simulink model "lab6_5"  (R2018b)
settings: Solver=VariableStepAuto  StartTime=0.0  StopTime=10.0  RelTol=1e-3
libraries: hdlsllib x17
settings Model: Creator=mllax8  LastModifiedBy=mllax8

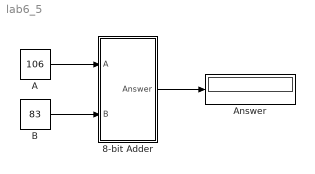
== system lab6_5 ==
  8-bit Adder : Subsystem
  A : Constant  Value=106  OutDataTypeStr=uint16
  Answer : Display
  B : Constant  Value=83  OutDataTypeStr=uint16
  wires:
  A/1 -> 8-bit Adder/1(A)
  B/1 -> 8-bit Adder/2(B)
  8-bit Adder/1(Answer) -> Answer/1

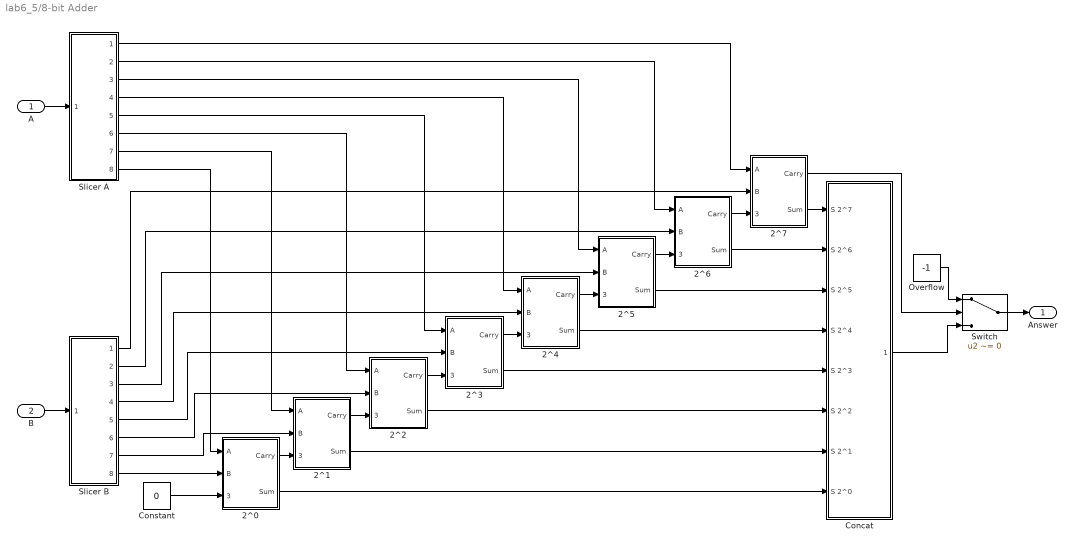
== system lab6_5/8-bit Adder ==
  A : Inport
  B : Inport  Port=2
  2^0 : Subsystem
  2^1 : Subsystem
  2^2 : Subsystem
  2^3 : Subsystem
  2^4 : Subsystem
  2^5 : Subsystem
  2^6 : Subsystem
  2^7 : Subsystem
  Concat : Subsystem
  Constant : Constant  Value=0
  Overflow : Constant  Value=-1  OutDataTypeStr=double
  Slicer A : Subsystem
  Slicer B : Subsystem
  Switch : Switch  Criteria=u2 ~= 0
  Answer : Outport
  wires:
  Slicer B/8("B 2^0 ") -> 2^0/2(B)
  2^7/2(Sum) -> Concat/1(S 2^7)
  Slicer B/5(B 2^3) -> 2^3/2(B)
  2^3/2(Sum) -> Concat/5(S 2^3)
  2^5/1(Carry) -> 2^6/3(Carry In)
  Slicer B/4(B 2^4) -> 2^4/2(B)
  Constant/1 -> 2^0/3(Carry In)
  2^4/2(Sum) -> Concat/4(S 2^4)
  Slicer B/6(B 2^2) -> 2^2/2(B)
  2^6/2(Sum) -> Concat/2(S 2^6)
  Slicer A/7(A 2^1) -> 2^1/1(A)
  2^4/1(Carry) -> 2^5/3(Carry In)
  2^5/2(Sum) -> Concat/3(S 2^5)
  2^3/1(Carry) -> 2^4/3(Carry In)
  Slicer B/1(B 2^7) -> 2^7/2(B)
  Slicer A/1(A 2^7) -> 2^7/1(A)
  2^1/1(Carry) -> 2^2/3(Carry In)
  2^0/1(Carry) -> 2^1/3(Carry In)
  Slicer B/3(B 2^5) -> 2^5/2(B)
  Slicer A/8("A 2^0 ") -> 2^0/1(A)
  2^0/2(Sum) -> Concat/8(S 2^0)
  Slicer A/5(A 2^3) -> 2^3/1(A)
  2^2/1(Carry) -> 2^3/3(Carry In)
  Slicer B/7(B 2^1) -> 2^1/2(B)
  Slicer A/4(A 2^4) -> 2^4/1(A)
  2^2/2(Sum) -> Concat/6(S 2^2)
  2^6/1(Carry) -> 2^7/3(Carry In)
  B/1 -> Slicer B/1(sign Int)
  Slicer A/2(A 2^6) -> 2^6/1(A)
  2^1/2(Sum) -> Concat/7(S 2^1)
  Slicer A/3(A 2^5) -> 2^5/1(A)
  Slicer B/2(B 2^6) -> 2^6/2(B)
  2^7/1(Carry) -> Switch/2
  Slicer A/6(A 2^2) -> 2^2/1(A)
  A/1 -> Slicer A/1(sign Int)
  Overflow/1 -> Switch/1
  Switch/1 -> Answer/1
  Concat/1(unsign Int) -> Switch/3

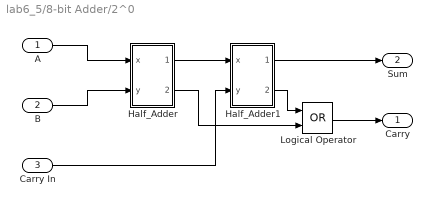
== system lab6_5/8-bit Adder/2^0 ==
  A : Inport
  B : Inport  Port=2
  Carry In : Inport  Port=3
  Half_Adder : Subsystem
  Half_Adder1 : Subsystem
  Logical Operator : Logic  Operator=OR  AllPortsSameDT=off  OutDataTypeStr=boolean
  Carry : Outport
  Sum : Outport  Port=2
  wires:
  Half_Adder1/1(Sum) -> Sum/1
  Carry In/1 -> Half_Adder1/2(y)
  Logical Operator/1 -> Carry/1
  Half_Adder1/2(Carry) -> Logical Operator/1
  A/1 -> Half_Adder/1(x)
  B/1 -> Half_Adder/2(y)
  Half_Adder/2(Carry) -> Logical Operator/2
  Half_Adder/1(Sum) -> Half_Adder1/1(x)

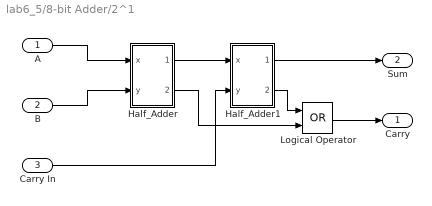
== system lab6_5/8-bit Adder/2^1 ==
  A : Inport
  B : Inport  Port=2
  Carry In : Inport  Port=3
  Half_Adder : Subsystem
  Half_Adder1 : Subsystem
  Logical Operator : Logic  Operator=OR  AllPortsSameDT=off  OutDataTypeStr=boolean
  Carry : Outport
  Sum : Outport  Port=2
  wires:
  Half_Adder1/1(Sum) -> Sum/1
  Carry In/1 -> Half_Adder1/2(y)
  Logical Operator/1 -> Carry/1
  Half_Adder1/2(Carry) -> Logical Operator/1
  A/1 -> Half_Adder/1(x)
  B/1 -> Half_Adder/2(y)
  Half_Adder/2(Carry) -> Logical Operator/2
  Half_Adder/1(Sum) -> Half_Adder1/1(x)

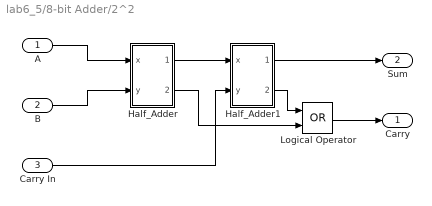
== system lab6_5/8-bit Adder/2^2 ==
  A : Inport
  B : Inport  Port=2
  Carry In : Inport  Port=3
  Half_Adder : Subsystem
  Half_Adder1 : Subsystem
  Logical Operator : Logic  Operator=OR  AllPortsSameDT=off  OutDataTypeStr=boolean
  Carry : Outport
  Sum : Outport  Port=2
  wires:
  Half_Adder1/1(Sum) -> Sum/1
  Carry In/1 -> Half_Adder1/2(y)
  Logical Operator/1 -> Carry/1
  Half_Adder1/2(Carry) -> Logical Operator/1
  A/1 -> Half_Adder/1(x)
  B/1 -> Half_Adder/2(y)
  Half_Adder/2(Carry) -> Logical Operator/2
  Half_Adder/1(Sum) -> Half_Adder1/1(x)

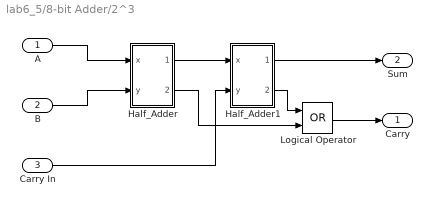
== system lab6_5/8-bit Adder/2^3 ==
  A : Inport
  B : Inport  Port=2
  Carry In : Inport  Port=3
  Half_Adder : Subsystem
  Half_Adder1 : Subsystem
  Logical Operator : Logic  Operator=OR  AllPortsSameDT=off  OutDataTypeStr=boolean
  Carry : Outport
  Sum : Outport  Port=2
  wires:
  Half_Adder1/1(Sum) -> Sum/1
  Carry In/1 -> Half_Adder1/2(y)
  Logical Operator/1 -> Carry/1
  Half_Adder1/2(Carry) -> Logical Operator/1
  A/1 -> Half_Adder/1(x)
  B/1 -> Half_Adder/2(y)
  Half_Adder/2(Carry) -> Logical Operator/2
  Half_Adder/1(Sum) -> Half_Adder1/1(x)

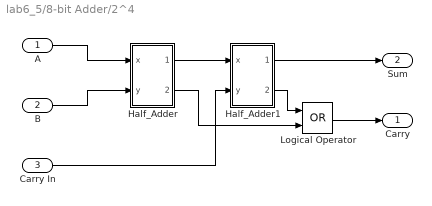
== system lab6_5/8-bit Adder/2^4 ==
  A : Inport
  B : Inport  Port=2
  Carry In : Inport  Port=3
  Half_Adder : Subsystem
  Half_Adder1 : Subsystem
  Logical Operator : Logic  Operator=OR  AllPortsSameDT=off  OutDataTypeStr=boolean
  Carry : Outport
  Sum : Outport  Port=2
  wires:
  Half_Adder1/1(Sum) -> Sum/1
  Carry In/1 -> Half_Adder1/2(y)
  Logical Operator/1 -> Carry/1
  Half_Adder1/2(Carry) -> Logical Operator/1
  A/1 -> Half_Adder/1(x)
  B/1 -> Half_Adder/2(y)
  Half_Adder/2(Carry) -> Logical Operator/2
  Half_Adder/1(Sum) -> Half_Adder1/1(x)

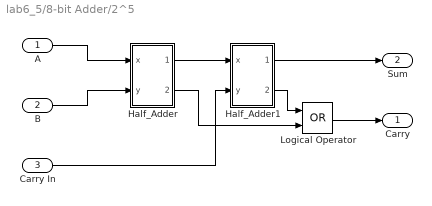
== system lab6_5/8-bit Adder/2^5 ==
  A : Inport
  B : Inport  Port=2
  Carry In : Inport  Port=3
  Half_Adder : Subsystem
  Half_Adder1 : Subsystem
  Logical Operator : Logic  Operator=OR  AllPortsSameDT=off  OutDataTypeStr=boolean
  Carry : Outport
  Sum : Outport  Port=2
  wires:
  Half_Adder1/1(Sum) -> Sum/1
  Carry In/1 -> Half_Adder1/2(y)
  Logical Operator/1 -> Carry/1
  Half_Adder1/2(Carry) -> Logical Operator/1
  A/1 -> Half_Adder/1(x)
  B/1 -> Half_Adder/2(y)
  Half_Adder/2(Carry) -> Logical Operator/2
  Half_Adder/1(Sum) -> Half_Adder1/1(x)

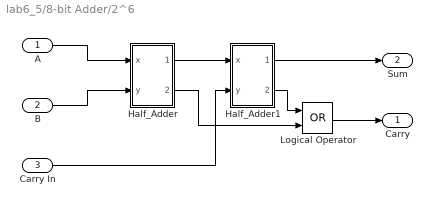
== system lab6_5/8-bit Adder/2^6 ==
  A : Inport
  B : Inport  Port=2
  Carry In : Inport  Port=3
  Half_Adder : Subsystem
  Half_Adder1 : Subsystem
  Logical Operator : Logic  Operator=OR  AllPortsSameDT=off  OutDataTypeStr=boolean
  Carry : Outport
  Sum : Outport  Port=2
  wires:
  Half_Adder1/1(Sum) -> Sum/1
  Carry In/1 -> Half_Adder1/2(y)
  Logical Operator/1 -> Carry/1
  Half_Adder1/2(Carry) -> Logical Operator/1
  A/1 -> Half_Adder/1(x)
  B/1 -> Half_Adder/2(y)
  Half_Adder/2(Carry) -> Logical Operator/2
  Half_Adder/1(Sum) -> Half_Adder1/1(x)

== system lab6_5/8-bit Adder/2^7 ==
  A : Inport
  B : Inport  Port=2
  Carry In : Inport  Port=3
  Half_Adder : Subsystem
  Half_Adder1 : Subsystem
  Logical Operator : Logic  Operator=OR  AllPortsSameDT=off  OutDataTypeStr=boolean
  Carry : Outport
  Sum : Outport  Port=2
  wires:
  Half_Adder1/1(Sum) -> Sum/1
  Carry In/1 -> Half_Adder1/2(y)
  Logical Operator/1 -> Carry/1
  Half_Adder1/2(Carry) -> Logical Operator/1
  A/1 -> Half_Adder/1(x)
  B/1 -> Half_Adder/2(y)
  Half_Adder/2(Carry) -> Logical Operator/2
  Half_Adder/1(Sum) -> Half_Adder1/1(x)

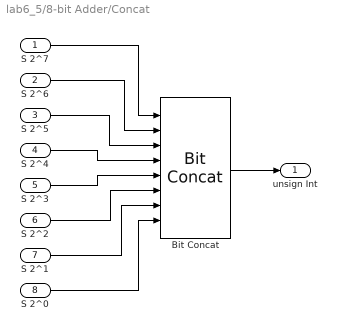
== system lab6_5/8-bit Adder/Concat ==
  S 2^7 : Inport
  S 2^6 : Inport  Port=2
  S 2^5 : Inport  Port=3
  S 2^4 : Inport  Port=4
  S 2^3 : Inport  Port=5
  S 2^2 : Inport  Port=6
  S 2^1 : Inport  Port=7
  S 2^0 : Inport  Port=8
  Bit Concat : hdlsllib/Logic and Bit Operations/Bit Concat  numInputs=8
      settings: SourceProductName=HDL Coder  SourceProductBaseCode=HD
  unsign Int : Outport
  wires:
  Bit Concat/1 -> unsign Int/1
  S 2^3/1 -> Bit Concat/5
  S 2^5/1 -> Bit Concat/3
  S 2^4/1 -> Bit Concat/4
  S 2^0/1 -> Bit Concat/8
  S 2^7/1 -> Bit Concat/1
  S 2^1/1 -> Bit Concat/7
  S 2^6/1 -> Bit Concat/2
  S 2^2/1 -> Bit Concat/6

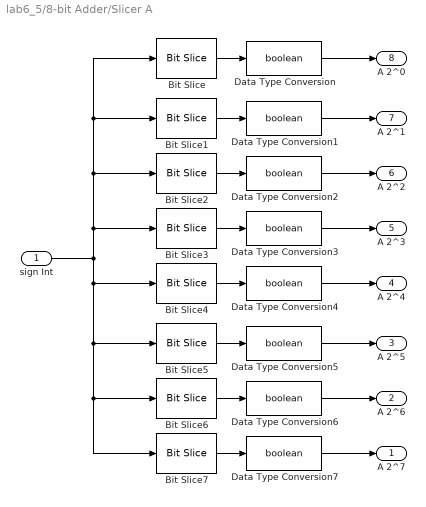
== system lab6_5/8-bit Adder/Slicer A ==
  sign Int : Inport  SampleTime=1
  Bit Slice : hdlsllib/Logic and Bit Operations/Bit Slice  lidx=0  ridx=0
  Bit Slice1 : hdlsllib/Logic and Bit Operations/Bit Slice  lidx=1  ridx=1
  Bit Slice2 : hdlsllib/Logic and Bit Operations/Bit Slice  lidx=2  ridx=2
  Bit Slice3 : hdlsllib/Logic and Bit Operations/Bit Slice  lidx=3  ridx=3
  Bit Slice4 : hdlsllib/Logic and Bit Operations/Bit Slice  lidx=4  ridx=4
  Bit Slice5 : hdlsllib/Logic and Bit Operations/Bit Slice  lidx=5  ridx=5
  Bit Slice6 : hdlsllib/Logic and Bit Operations/Bit Slice  lidx=6  ridx=6
  Bit Slice7 : hdlsllib/Logic and Bit Operations/Bit Slice  lidx=7  ridx=7
  Data Type Conversion{,1..7} (8 alike) : DataTypeConversion  OutDataTypeStr=boolean
  A 2^7 : Outport
  A 2^6 : Outport  Port=2
  A 2^5 : Outport  Port=3
  A 2^4 : Outport  Port=4
  A 2^3 : Outport  Port=5
  A 2^2 : Outport  Port=6
  A 2^1 : Outport  Port=7
  "A 2^0 " : Outport  Port=8
  wires:
  Data Type Conversion/1 -> "A 2^0 "/1
  Data Type Conversion5/1 -> A 2^5/1
  Bit Slice1/1 -> Data Type Conversion1/1
  Bit Slice5/1 -> Data Type Conversion5/1
  Bit Slice7/1 -> Data Type Conversion7/1
  Bit Slice2/1 -> Data Type Conversion2/1
  Bit Slice3/1 -> Data Type Conversion3/1
  Data Type Conversion6/1 -> A 2^6/1
  Bit Slice4/1 -> Data Type Conversion4/1
  sign Int/1 -> Bit Slice4/1, Bit Slice5/1, Bit Slice6/1, Bit Slice7/1, Bit Slice3/1, Bit Slice2/1, Bit Slice1/1, Bit Slice/1
  Data Type Conversion1/1 -> A 2^1/1
  Data Type Conversion2/1 -> A 2^2/1
  Bit Slice/1 -> Data Type Conversion/1
  Bit Slice6/1 -> Data Type Conversion6/1
  Data Type Conversion3/1 -> A 2^3/1
  Data Type Conversion4/1 -> A 2^4/1
  Data Type Conversion7/1 -> A 2^7/1

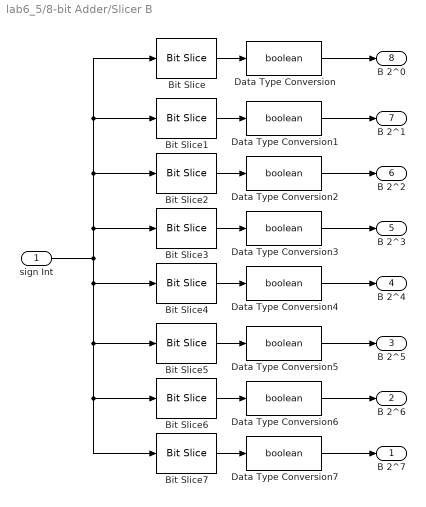
== system lab6_5/8-bit Adder/Slicer B ==
  sign Int : Inport  SampleTime=1
  Bit Slice : hdlsllib/Logic and Bit Operations/Bit Slice  lidx=0  ridx=0
  Bit Slice1 : hdlsllib/Logic and Bit Operations/Bit Slice  lidx=1  ridx=1
  Bit Slice2 : hdlsllib/Logic and Bit Operations/Bit Slice  lidx=2  ridx=2
  Bit Slice3 : hdlsllib/Logic and Bit Operations/Bit Slice  lidx=3  ridx=3
  Bit Slice4 : hdlsllib/Logic and Bit Operations/Bit Slice  lidx=4  ridx=4
  Bit Slice5 : hdlsllib/Logic and Bit Operations/Bit Slice  lidx=5  ridx=5
  Bit Slice6 : hdlsllib/Logic and Bit Operations/Bit Slice  lidx=6  ridx=6
  Bit Slice7 : hdlsllib/Logic and Bit Operations/Bit Slice  lidx=7  ridx=7
  Data Type Conversion{,1..7} (8 alike) : DataTypeConversion  OutDataTypeStr=boolean
  B 2^7 : Outport
  B 2^6 : Outport  Port=2
  B 2^5 : Outport  Port=3
  B 2^4 : Outport  Port=4
  B 2^3 : Outport  Port=5
  B 2^2 : Outport  Port=6
  B 2^1 : Outport  Port=7
  "B 2^0 " : Outport  Port=8
  wires:
  Data Type Conversion/1 -> "B 2^0 "/1
  Data Type Conversion5/1 -> B 2^5/1
  Bit Slice1/1 -> Data Type Conversion1/1
  Bit Slice5/1 -> Data Type Conversion5/1
  Bit Slice7/1 -> Data Type Conversion7/1
  Bit Slice2/1 -> Data Type Conversion2/1
  Bit Slice3/1 -> Data Type Conversion3/1
  Data Type Conversion6/1 -> B 2^6/1
  Bit Slice4/1 -> Data Type Conversion4/1
  sign Int/1 -> Bit Slice4/1, Bit Slice5/1, Bit Slice6/1, Bit Slice7/1, Bit Slice3/1, Bit Slice2/1, Bit Slice1/1, Bit Slice/1
  Data Type Conversion1/1 -> B 2^1/1
  Data Type Conversion2/1 -> B 2^2/1
  Bit Slice/1 -> Data Type Conversion/1
  Bit Slice6/1 -> Data Type Conversion6/1
  Data Type Conversion3/1 -> B 2^3/1
  Data Type Conversion4/1 -> B 2^4/1
  Data Type Conversion7/1 -> B 2^7/1

== system lab6_5/8-bit Adder/2^0/Half_Adder ==
  x : Inport
  y : Inport  Port=2
  Calc Carry : Logic  AllPortsSameDT=off  OutDataTypeStr=boolean
  Calc Sum : Logic  Operator=XOR  AllPortsSameDT=off  OutDataTypeStr=boolean
  Sum : Outport
  Carry : Outport  Port=2
  wires:
  Calc Carry/1 -> Carry/1
  x/1 -> Calc Carry/1, Calc Sum/1
  Calc Sum/1 -> Sum/1
  y/1 -> Calc Sum/2, Calc Carry/2

== system lab6_5/8-bit Adder/2^0/Half_Adder1 ==
  x : Inport
  y : Inport  Port=2
  Calc Carry : Logic  AllPortsSameDT=off  OutDataTypeStr=boolean
  Calc Sum : Logic  Operator=XOR  AllPortsSameDT=off  OutDataTypeStr=boolean
  Sum : Outport
  Carry : Outport  Port=2
  wires:
  Calc Carry/1 -> Carry/1
  x/1 -> Calc Carry/1, Calc Sum/1
  Calc Sum/1 -> Sum/1
  y/1 -> Calc Sum/2, Calc Carry/2

== system lab6_5/8-bit Adder/2^1/Half_Adder ==
  x : Inport
  y : Inport  Port=2
  Calc Carry : Logic  AllPortsSameDT=off  OutDataTypeStr=boolean
  Calc Sum : Logic  Operator=XOR  AllPortsSameDT=off  OutDataTypeStr=boolean
  Sum : Outport
  Carry : Outport  Port=2
  wires:
  Calc Carry/1 -> Carry/1
  x/1 -> Calc Carry/1, Calc Sum/1
  Calc Sum/1 -> Sum/1
  y/1 -> Calc Sum/2, Calc Carry/2

== system lab6_5/8-bit Adder/2^1/Half_Adder1 ==
  x : Inport
  y : Inport  Port=2
  Calc Carry : Logic  AllPortsSameDT=off  OutDataTypeStr=boolean
  Calc Sum : Logic  Operator=XOR  AllPortsSameDT=off  OutDataTypeStr=boolean
  Sum : Outport
  Carry : Outport  Port=2
  wires:
  Calc Carry/1 -> Carry/1
  x/1 -> Calc Carry/1, Calc Sum/1
  Calc Sum/1 -> Sum/1
  y/1 -> Calc Sum/2, Calc Carry/2

== system lab6_5/8-bit Adder/2^2/Half_Adder ==
  x : Inport
  y : Inport  Port=2
  Calc Carry : Logic  AllPortsSameDT=off  OutDataTypeStr=boolean
  Calc Sum : Logic  Operator=XOR  AllPortsSameDT=off  OutDataTypeStr=boolean
  Sum : Outport
  Carry : Outport  Port=2
  wires:
  Calc Carry/1 -> Carry/1
  x/1 -> Calc Carry/1, Calc Sum/1
  Calc Sum/1 -> Sum/1
  y/1 -> Calc Sum/2, Calc Carry/2

== system lab6_5/8-bit Adder/2^2/Half_Adder1 ==
  x : Inport
  y : Inport  Port=2
  Calc Carry : Logic  AllPortsSameDT=off  OutDataTypeStr=boolean
  Calc Sum : Logic  Operator=XOR  AllPortsSameDT=off  OutDataTypeStr=boolean
  Sum : Outport
  Carry : Outport  Port=2
  wires:
  Calc Carry/1 -> Carry/1
  x/1 -> Calc Carry/1, Calc Sum/1
  Calc Sum/1 -> Sum/1
  y/1 -> Calc Sum/2, Calc Carry/2

== system lab6_5/8-bit Adder/2^3/Half_Adder ==
  x : Inport
  y : Inport  Port=2
  Calc Carry : Logic  AllPortsSameDT=off  OutDataTypeStr=boolean
  Calc Sum : Logic  Operator=XOR  AllPortsSameDT=off  OutDataTypeStr=boolean
  Sum : Outport
  Carry : Outport  Port=2
  wires:
  Calc Carry/1 -> Carry/1
  x/1 -> Calc Carry/1, Calc Sum/1
  Calc Sum/1 -> Sum/1
  y/1 -> Calc Sum/2, Calc Carry/2

== system lab6_5/8-bit Adder/2^3/Half_Adder1 ==
  x : Inport
  y : Inport  Port=2
  Calc Carry : Logic  AllPortsSameDT=off  OutDataTypeStr=boolean
  Calc Sum : Logic  Operator=XOR  AllPortsSameDT=off  OutDataTypeStr=boolean
  Sum : Outport
  Carry : Outport  Port=2
  wires:
  Calc Carry/1 -> Carry/1
  x/1 -> Calc Carry/1, Calc Sum/1
  Calc Sum/1 -> Sum/1
  y/1 -> Calc Sum/2, Calc Carry/2

== system lab6_5/8-bit Adder/2^4/Half_Adder ==
  x : Inport
  y : Inport  Port=2
  Calc Carry : Logic  AllPortsSameDT=off  OutDataTypeStr=boolean
  Calc Sum : Logic  Operator=XOR  AllPortsSameDT=off  OutDataTypeStr=boolean
  Sum : Outport
  Carry : Outport  Port=2
  wires:
  Calc Carry/1 -> Carry/1
  x/1 -> Calc Carry/1, Calc Sum/1
  Calc Sum/1 -> Sum/1
  y/1 -> Calc Sum/2, Calc Carry/2

== system lab6_5/8-bit Adder/2^4/Half_Adder1 ==
  x : Inport
  y : Inport  Port=2
  Calc Carry : Logic  AllPortsSameDT=off  OutDataTypeStr=boolean
  Calc Sum : Logic  Operator=XOR  AllPortsSameDT=off  OutDataTypeStr=boolean
  Sum : Outport
  Carry : Outport  Port=2
  wires:
  Calc Carry/1 -> Carry/1
  x/1 -> Calc Carry/1, Calc Sum/1
  Calc Sum/1 -> Sum/1
  y/1 -> Calc Sum/2, Calc Carry/2

== system lab6_5/8-bit Adder/2^5/Half_Adder ==
  x : Inport
  y : Inport  Port=2
  Calc Carry : Logic  AllPortsSameDT=off  OutDataTypeStr=boolean
  Calc Sum : Logic  Operator=XOR  AllPortsSameDT=off  OutDataTypeStr=boolean
  Sum : Outport
  Carry : Outport  Port=2
  wires:
  Calc Carry/1 -> Carry/1
  x/1 -> Calc Carry/1, Calc Sum/1
  Calc Sum/1 -> Sum/1
  y/1 -> Calc Sum/2, Calc Carry/2

== system lab6_5/8-bit Adder/2^5/Half_Adder1 ==
  x : Inport
  y : Inport  Port=2
  Calc Carry : Logic  AllPortsSameDT=off  OutDataTypeStr=boolean
  Calc Sum : Logic  Operator=XOR  AllPortsSameDT=off  OutDataTypeStr=boolean
  Sum : Outport
  Carry : Outport  Port=2
  wires:
  Calc Carry/1 -> Carry/1
  x/1 -> Calc Carry/1, Calc Sum/1
  Calc Sum/1 -> Sum/1
  y/1 -> Calc Sum/2, Calc Carry/2

== system lab6_5/8-bit Adder/2^6/Half_Adder ==
  x : Inport
  y : Inport  Port=2
  Calc Carry : Logic  AllPortsSameDT=off  OutDataTypeStr=boolean
  Calc Sum : Logic  Operator=XOR  AllPortsSameDT=off  OutDataTypeStr=boolean
  Sum : Outport
  Carry : Outport  Port=2
  wires:
  Calc Carry/1 -> Carry/1
  x/1 -> Calc Carry/1, Calc Sum/1
  Calc Sum/1 -> Sum/1
  y/1 -> Calc Sum/2, Calc Carry/2

== system lab6_5/8-bit Adder/2^6/Half_Adder1 ==
  x : Inport
  y : Inport  Port=2
  Calc Carry : Logic  AllPortsSameDT=off  OutDataTypeStr=boolean
  Calc Sum : Logic  Operator=XOR  AllPortsSameDT=off  OutDataTypeStr=boolean
  Sum : Outport
  Carry : Outport  Port=2
  wires:
  Calc Carry/1 -> Carry/1
  x/1 -> Calc Carry/1, Calc Sum/1
  Calc Sum/1 -> Sum/1
  y/1 -> Calc Sum/2, Calc Carry/2

== system lab6_5/8-bit Adder/2^7/Half_Adder ==
  x : Inport
  y : Inport  Port=2
  Calc Carry : Logic  AllPortsSameDT=off  OutDataTypeStr=boolean
  Calc Sum : Logic  Operator=XOR  AllPortsSameDT=off  OutDataTypeStr=boolean
  Sum : Outport
  Carry : Outport  Port=2
  wires:
  Calc Carry/1 -> Carry/1
  x/1 -> Calc Carry/1, Calc Sum/1
  Calc Sum/1 -> Sum/1
  y/1 -> Calc Sum/2, Calc Carry/2

== system lab6_5/8-bit Adder/2^7/Half_Adder1 ==
  x : Inport
  y : Inport  Port=2
  Calc Carry : Logic  AllPortsSameDT=off  OutDataTypeStr=boolean
  Calc Sum : Logic  Operator=XOR  AllPortsSameDT=off  OutDataTypeStr=boolean
  Sum : Outport
  Carry : Outport  Port=2
  wires:
  Calc Carry/1 -> Carry/1
  x/1 -> Calc Carry/1, Calc Sum/1
  Calc Sum/1 -> Sum/1
  y/1 -> Calc Sum/2, Calc Carry/2
